simulink model "Assignment_TestGen10"  (R2017b)
settings: Solver=FixedStepDiscrete  StartTime=0.0  StopTime=10.0  RelTol=1e-3
settings Model: Creator=hbourbou  LastModifiedBy=hbourbou
settings DebuggingCC: ParameterOverflowMsg=none

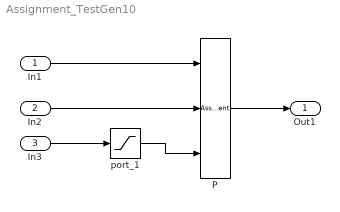
== system Assignment_TestGen10 ==
  In1 : Inport  OutDataTypeStr=int16  PortDimensions=[3 3]
  In2 : Inport  Port=2  OutDataTypeStr=int16  PortDimensions=[2 3]
  In3 : Inport  Port=3  OutMin=0  OutMax=1
  P : Assignment  NumberOfDimensions=2  IndexMode=Zero-based  DiagnosticForDimensions=Warning  IndexOptions=Starting index (port),Assign all  Indices=[],[]  OutputSizes=,
  port_1 : Saturate  UpperLimit=1  LowerLimit=0
  Out1 : Outport
  wires:
  In1/1 -> P/1
  In2/1 -> P/2
  port_1/1 -> P/3
  In3/1 -> port_1/1
  P/1 -> Out1/1
